simulink model "Temp_Control"  (R2019b)
settings: Solver=ode8  StartTime=0.0  StopTime=5  RelTol=1e-3  EnableMultiTasking=on
libraries: arduinolib x7, dspfdesign x2
settings Model: SimulationMode=external  SILPILModeSetting=veronly  PacingRate=0.220000  ExtModeTrigDuration=2  Creator=Bryan  LastModifiedBy=Bryan
settings OptimizationCC: EnhancedBackFolding=on  PassReuseOutputArgsAs=Individual arguments  MaxStackSize=64  OptimizeBlockOrder=speed  DifferentSizesBufferReuse=on  OptimizationCustomize=off  EfficientTunableParamExpr=on
settings DebuggingCC: ParameterPrecisionLossMsg=none  ParameterTunabilityLossMsg=error
settings HardwareCC: ProdBitPerInt=16  ProdBitPerPointer=16  ProdBitPerSizeT=16  ProdBitPerPtrDiffT=16  ProdLargestAtomicFloat=None  ProdWordSize=8  ProdHWDeviceType=Atmel->AVR  UseEmbeddedCoderFeatures=off
settings SFSimCC: MATLABDynamicMemAlloc=off
settings RTWCC: SystemTargetFile=ert.tlc  HardwareBoard=Arduino Uno  TLCOptions=-aInlineSetEventsForThisBaseRateFcn=TLC_FALSE -aSuppressMultiTaskScheduler=TLC_FALSE -aRateBasedStepFcn=1  TemplateMakefile=ert_default_tmf  GenerateReport=on  Toolchain=Arduino AVR  IncludeHyperlinkInReport=on  LaunchReport=on  GenerateTraceInfo=on  GenerateTraceReport=on  GenerateTraceReportSl=on  GenerateTraceReportSf=on  GenerateTraceReportEml=on
settings CodeAppCC: ForceParamTrailComments=on  IgnoreCustomStorageClasses=off  OperatorAnnotations=on  SimulinkDataObjDesc=on  SFDataObjDesc=on  InsertBlockDesc=on
settings ERTTargetCC: TargetLangStandard=C99 (ISO)  SupportContinuousTime=on  SupportNonInlinedSFcns=on  SupportVariableSizeSignals=on  ExtModeStaticAllocSize=250  RootIOFormat=Structure reference

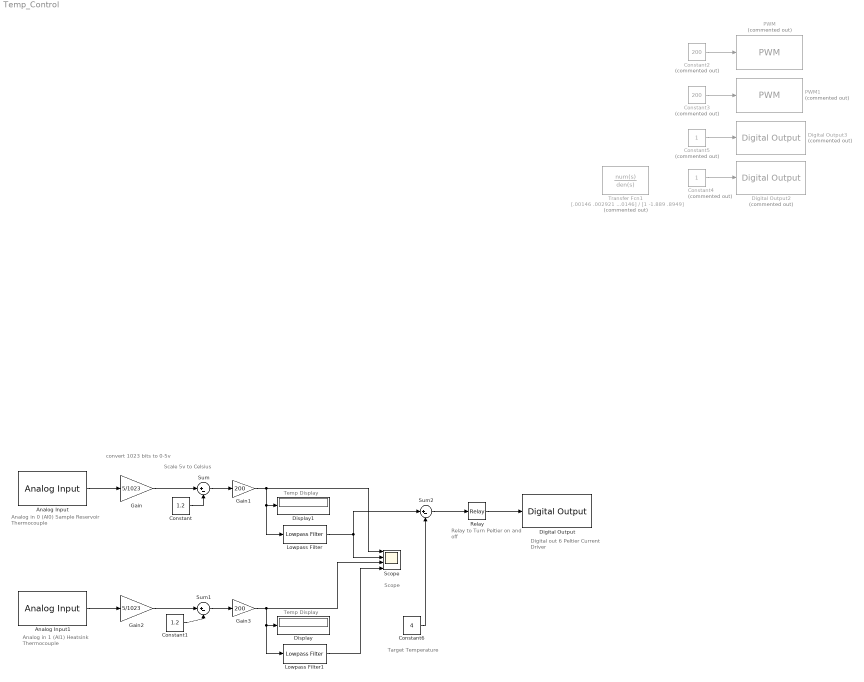
== system Temp_Control ==
  note: Digital out 6
      | Peltier Current Driver
  note: Relay to Turn Peltier
      | on and off
  note: Target Temperature
  note: Scope
  note: Temp Display
  note: Scale 5v to Celsius
  note: convert 1023 bits to 0-5v
  note: Analog in 0 (AI0)
      | Sample Reservoir Thermocouple
  note: Analog in 1 (AI1)
      | Heatsink Thermocouple
  note: Temp Display
  Analog Input : arduinolib/Analog Input  pinNumber=0  ReadResultsOnly=off  ConversionTriggerSource=Software  ExternalTriggerType=uint32(0)  OutputDataType=uint16  EnableConversionCompleteNotify=off  EnableOuputStatus=off  SampleTime=-1  blockPlatform=arduino
  Analog Input1 : arduinolib/Analog Input  pinNumber=1  ReadResultsOnly=off  ConversionTriggerSource=Software  ExternalTriggerType=uint32(0)  OutputDataType=uint16  EnableConversionCompleteNotify=off  EnableOuputStatus=off  SampleTime=-1  blockPlatform=arduino
  Constant : Constant  Value=1.2
  Constant1 : Constant  Value=1.2
  Constant2 : Constant  Commented=on  Value=200
  Constant3 : Constant  Commented=on  Value=200
  Constant4 : Constant  Commented=on
  Constant5 : Constant  Commented=on
  Constant6 : Constant  Value=4
  Digital Output : arduinolib/Digital Output  pinNumber=6  blockPlatform=arduino
  Digital Output2 : arduinolib/Digital Output  Commented=on  pinNumber=2  blockPlatform=arduino
  Digital Output3 : arduinolib/Digital Output  Commented=on  pinNumber=11  blockPlatform=arduino
  Display : Display
  Display1 : Display
  Gain : Gain  Gain=5/1023
  Gain1 : Gain  Gain=200
  Gain2 : Gain  Gain=5/1023
  Gain3 : Gain  Gain=200
  Lowpass Filter : dspfdesign/Lowpass Filter  FilterType=FIR  DesignForMinimumOrder=on  FilterOrder=50  PassbandFrequency=50  StopbandFrequency=1000  PassbandRipple=0.1  StopbandAttenuation=80  InheritSampleRate=off  SampleRate=44100  SimulateUsing=Interpreted execution  roundingMode=Floor  coeffsDataTypeStr=fixdt(1,16)
  Lowpass Filter1 : dspfdesign/Lowpass Filter  FilterType=FIR  DesignForMinimumOrder=on  FilterOrder=50  PassbandFrequency=50  StopbandFrequency=1000  PassbandRipple=0.1  StopbandAttenuation=80  InheritSampleRate=off  SampleRate=44100  SimulateUsing=Interpreted execution  roundingMode=Floor  coeffsDataTypeStr=fixdt(1,16)
  PWM : arduinolib/PWM  Commented=on  pinNumber=6  EnableInputFrequency=off  InitialFrequency=2000  InitialDutyCycle=0  NotificationType=None  blockPlatform=arduino
  PWM1 : arduinolib/PWM  Commented=on  pinNumber=5  EnableInputFrequency=off  InitialFrequency=2000  InitialDutyCycle=0  NotificationType=None  blockPlatform=arduino
  Relay : Relay  OnSwitchValue=30  OffSwitchValue=0
  Scope : Scope  NumInputPorts=4
  Sum : Sum  Inputs=|+-
  Sum1 : Sum  Inputs=|+-
  Sum2 : Sum  Inputs=|+-
  Transfer Fcn1 : TransferFcn  Commented=on  Numerator=[.00146 .002921 .00146]  Denominator=[1 -1.889 .8949]
  wires:
  Relay/1 -> Digital Output/1
  Analog Input/1 -> Gain/1
  Constant1/1 -> Sum1/2
  Gain3/1 -> Lowpass Filter1/1, Display/1, Scope/3
  Sum/1 -> Gain1/1
  Constant2/1 -> PWM/1
  Constant/1 -> Sum/2
  Constant3/1 -> PWM1/1
  Sum1/1 -> Gain3/1
  Constant4/1 -> Digital Output2/1
  Lowpass Filter/1 -> Scope/2, Sum2/1
  Gain/1 -> Sum/1
  Constant5/1 -> Digital Output3/1
  Analog Input1/1 -> Gain2/1
  Gain2/1 -> Sum1/1
  Gain1/1 -> Lowpass Filter/1, Display1/1, Scope/1
  Lowpass Filter1/1 -> Scope/4
  Sum2/1 -> Relay/1
  Constant6/1 -> Sum2/2
